simulink subsystem "subsys_dynamic_plaque"  (R2021a)
settings: Solver=VariableStepAuto  StartTime=0.0  StopTime=10.0  RelTol=1e-3
values from neighbouring files (symbols this model uses):
  Fg = mp*g    (= 4.33602)    [dynamic_plaque.m]
  Jp = 1.347    [dynamic_plaque.m]
  mp = 0.442    [dynamic_plaque.m]
  Xa = r_abc    (= 0.0952)    [Hauteur_Aimants_Plaque.m]    (also in dynamic_plaque.m)
  Xb = -r_abc*sin(deg2rad(30))    [Hauteur_Aimants_Plaque.m]    (also in dynamic_plaque.m = -r*sin(deg2rad(30)))
  Xc = -r_abc*sin(deg2rad(30))    [Hauteur_Aimants_Plaque.m]    (also in dynamic_plaque.m = -r*sin(deg2rad(30)))
  Ya = 0    [Hauteur_Aimants_Plaque.m]    (also in dynamic_plaque.m)
  Yb = r_abc*cos(deg2rad(30))    [Hauteur_Aimants_Plaque.m]    (also in dynamic_plaque.m = r*cos(deg2rad(30)))
  Yc = -r_abc*cos(deg2rad(30))    [Hauteur_Aimants_Plaque.m]    (also in dynamic_plaque.m = -r*cos(deg2rad(30)))
settings Model: Creator=antho  LastModifiedBy=dupa1607

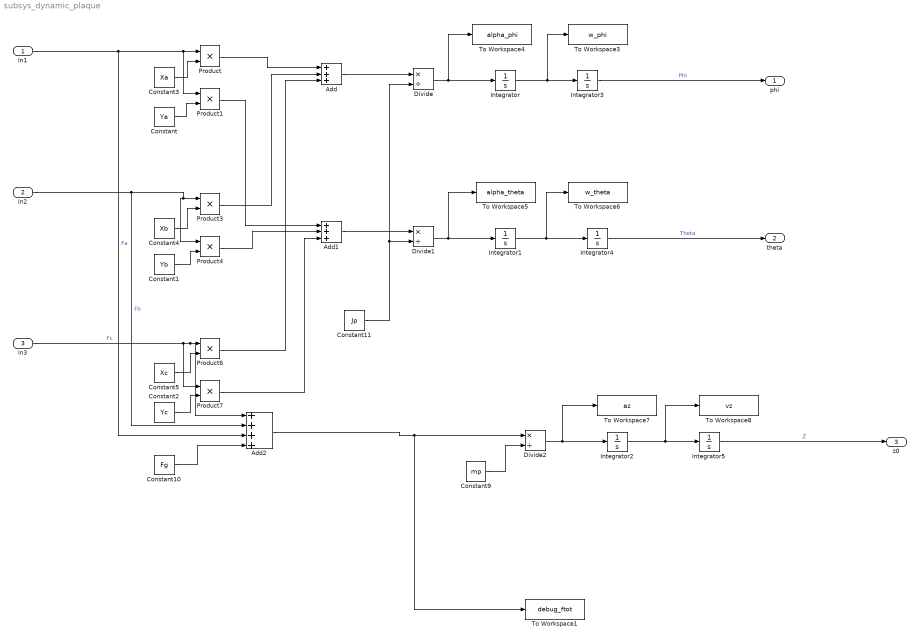
== system subsys_dynamic_plaque ==
  In1 : Inport
  In2 : Inport  Port=2
  In3 : Inport  Port=3
  Add : Sum  Inputs=+++
  Add1 : Sum  Inputs=+++
  Add2 : Sum  Inputs=++++
  Constant : Constant  Value=Ya
  Constant1 : Constant  Value=Yb
  Constant10 : Constant  Value=Fg
  Constant11 : Constant  Value=Jp
  Constant2 : Constant  Value=Yc
  Constant3 : Constant  Value=Xa
  Constant4 : Constant  Value=Xb
  Constant5 : Constant  Value=Xc
  Constant9 : Constant  Value=mp
  Divide : Product  Inputs=*/
  Divide1 : Product  Inputs=*/
  Divide2 : Product  Inputs=*/
  Integrator{,1..5} (6 alike) : Integrator
  Product{,1,3..4,6..7} (6 alike) : Product
  To Workspace1 : ToWorkspace  VariableName=debug_ftot  SaveFormat=Timeseries  SampleTime=-1
  To Workspace3 : ToWorkspace  VariableName=w_phi  SaveFormat=Timeseries  SampleTime=-1
  To Workspace4 : ToWorkspace  VariableName=alpha_phi  SaveFormat=Timeseries  SampleTime=-1
  To Workspace5 : ToWorkspace  VariableName=alpha_theta  SaveFormat=Timeseries  SampleTime=-1
  To Workspace6 : ToWorkspace  VariableName=w_theta  SaveFormat=Timeseries  SampleTime=-1
  To Workspace7 : ToWorkspace  VariableName=az  SaveFormat=Timeseries  SampleTime=-1
  To Workspace8 : ToWorkspace  VariableName=vz  SaveFormat=Timeseries  SampleTime=-1
  phi : Outport
  theta : Outport  Port=2
  z0 : Outport  Port=3
  wires:
  Product/1 -> Add/1
  Constant5/1 -> Product6/2
  Integrator/1 -> To Workspace3/1, Integrator3/1
  Constant2/1 -> Product7/2
  Product3/1 -> Add/2
  Add1/1 -> Divide1/1
  Constant/1 -> Product1/2
  Integrator3/1 -> phi/1  "Phi"
  Constant3/1 -> Product/2
  Product6/1 -> Add/3
  Divide/1 -> To Workspace4/1, Integrator/1
  Constant1/1 -> Product4/2
  Add/1 -> Divide/1
  Product1/1 -> Add1/1
  Divide2/1 -> To Workspace7/1, Integrator2/1
  Product4/1 -> Add1/2
  Constant9/1 -> Divide2/2
  Constant4/1 -> Product3/2
  Integrator5/1 -> z0/1  "Z"
  Integrator4/1 -> theta/1  "Theta"
  Integrator2/1 -> To Workspace8/1, Integrator5/1
  In3/1 -> Product7/1, Product6/1, Add2/1  "Fc"
  Product7/1 -> Add1/3
  Integrator1/1 -> To Workspace6/1, Integrator4/1
  Divide1/1 -> To Workspace5/1, Integrator1/1
  In2/1 -> Product3/1, Product4/1, Add2/2  "Fb"
  In1/1 -> Product1/1, Product/1, Add2/3  "Fa"
  Constant11/1 -> Divide1/2, Divide/2
  Constant10/1 -> Add2/4
  Add2/1 -> Divide2/1, To Workspace1/1
